simulink model "phasor08_ieee13_1_sm_master"  (Simulink 10.2)
settings: Solver=ode4  StartTime=0.0  StopTime=inf  FixedStep=0.01  RelTol=1e-3  EnableMultiTasking=on
PreLoadFcn:
  | Ts=0.01;
PostLoadFcn:
  | Ts=0.01;
InitFcn:
  | Ts=0.01;
StartFcn:
  | Ts=0.01;
libraries: opal_lib x5, eph_overcurrent x1, rtlab_phasor x1
settings Model: Creator=ZhiqiZhao  LastModifiedBy=xjk374
settings DataIOCC: LimitDataPoints=on
settings OptimizationCC: ExpressionDepthLimit=2147483647  LocalBlockOutputs=off
settings DebuggingCC: SolverPrmCheckMsg=warning  AllowSymbolicDim=off  StateNameClashWarn=warning
settings RTWCC: GenCodeOnly=on

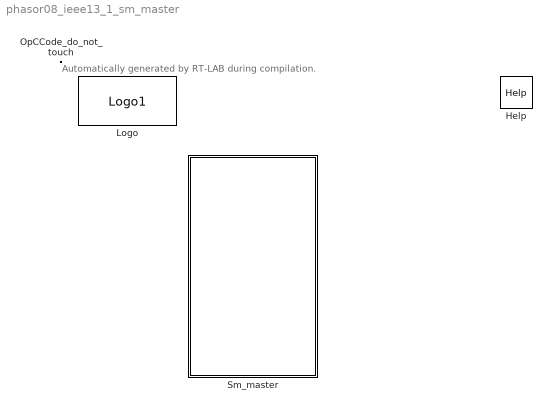
== system phasor08_ieee13_1_sm_master ==
  note: Automatically generated by RT-LAB during compilation.
  Help : opal_lib/Help  docfile=../help/ePH_IEEE13.html
  Logo : opal_lib/Logo1  vide=[]
  OpCCode_do_not_touch : opal_lib/Communication/OpCCode  SystemSampleTime=-1  VariantActivationTime=update diagram  Latency=0  AutoFrameSizeCalculation=off
  Sm_master : Subsystem

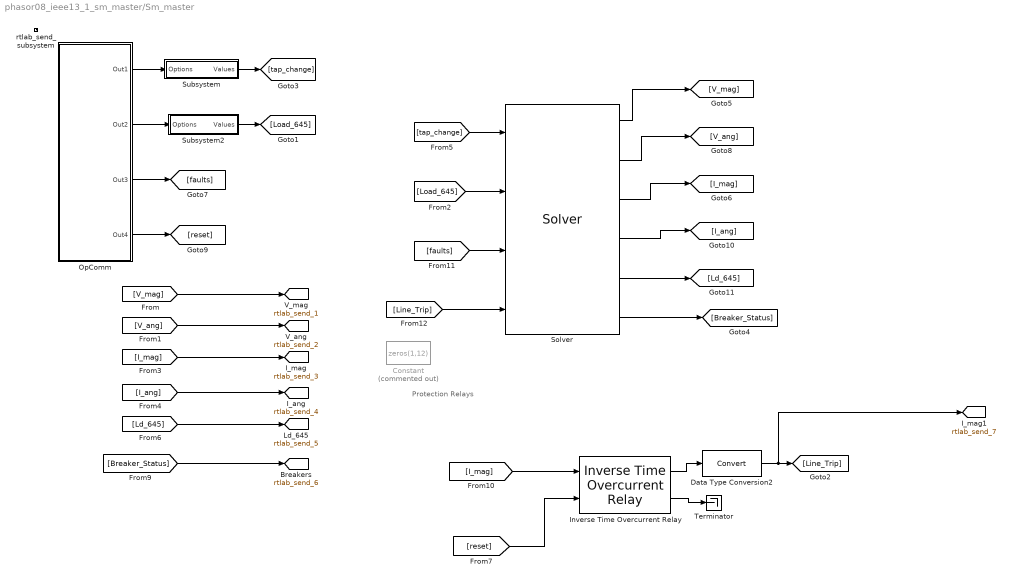
== system phasor08_ieee13_1_sm_master/Sm_master ==
  note: Protection
      | Relays
  Constant : Constant  Commented=on  Value=zeros(1,12)
  Data Type Conversion2 : DataTypeConversion
  Inverse Time Overcurrent Relay : eph_overcurrent/Inverse Time Overcurrent Relay  Ts=Ts  N=12  characteristic=6: I.E.C Class A - Standard inverse (0, 0.14, 0.02)  Ipck_51P=1000*ones(1,12)  TD51P=0.05*ones(1,12)
  OpComm : Subsystem
      mask init:
      | opmaskdisplay('maskdisplay_block',gcb,'disp(''OpComm'')');
      mask Display:
      | patch([0 0.5 0.7 0],[1 1 0 0],[0.7 0.75 0.9]);
      | patch([1 0.53 0.73 1],[1 1 0 0],[1 0.8 0.7]);
      | plot([0 0 1 1 0],[0 1 1 0 0]);
      | disp('OpComm')
  Solver : rtlab_phasor/Solver  epname=System  extension=Excel  use_udb=off  xls='phasor08_IEEE13.xls'  raw='4992b.raw'  dyr='4992b.dyr'  fmu2builtin=off  cyme='ieee13.sxst'  cyme_pf=''  cyme_unbalanced=on  powerfactory='network.xml'  builtin=on  lazy_netlist=on  capidir='CAPI'  fmudir=''  capiprefix=capicomp_  fmuprefix=fmucomp_  logging=off  sim_mode=Dynamic simulation only (without power-flow)  dt=Ts  pf_init_method=From input data  pf_tol_v=0.000001  pf_max_it=100  pf_smart_start=off  pf_flat_start=off  pf_export=off  pfrequest=off  pf_then_dyn=off  np=1  exporty=off  optim_threads=off  perflog_on=off  script_activate_postinit=off  script_postinit_name=''
  Subsystem : Subsystem
  Subsystem2 : Subsystem
  Terminator : Terminator
  rtlab_send_subsystem : Subsystem  Priority=-100
      mask Display: text(0,0,'');
  tag scope: rtlab_send_1=global, rtlab_send_2=global, rtlab_send_3=global, rtlab_send_4=global, rtlab_send_5=global, rtlab_send_6=global, rtlab_send_7=global
  wires:
  [tap_change] -> Solver/1
  Solver/1 -> [V_mag]
  Solver/2 -> [V_ang]
  Solver/3 -> [I_mag]
  Solver/4 -> [I_ang]
  Solver/5 -> [Ld_645]
  [Load_645] -> Solver/2
  [V_mag] -> [rtlab_send_1]
  [V_ang] -> [rtlab_send_2]
  [I_ang] -> [rtlab_send_4]
  [I_mag] -> [rtlab_send_3]
  [Ld_645] -> [rtlab_send_5]
  OpComm/1(Out1) -> Subsystem/1(Options)
  OpComm/2(Out2) -> Subsystem2/1(Options)
  Subsystem/1(Values) -> [tap_change]
  Subsystem2/1(Values) -> [Load_645]
  Inverse Time Overcurrent Relay/2 -> Terminator/1
  [reset] -> Inverse Time Overcurrent Relay/2
  Data Type Conversion2/1 -> [rtlab_send_7], [Line_Trip]
  Solver/6 -> [Breaker_Status]
  [Breaker_Status] -> [rtlab_send_6]
  Inverse Time Overcurrent Relay/1 -> Data Type Conversion2/1
  [I_mag] -> Inverse Time Overcurrent Relay/1
  OpComm/3(Out3) -> [faults]
  [faults] -> Solver/3
  [Line_Trip] -> Solver/4
  OpComm/4(Out4) -> [reset]

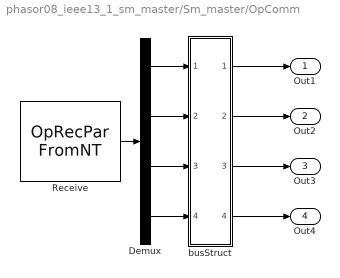
== system phasor08_ieee13_1_sm_master/Sm_master/OpComm ==
  Demux : Demux  Outputs="[7  5  4  1]"
  Receive : opal_lib/Communication/OpRecPar FromNT  Data_width=17  InitialConditions=[8;8;8;1;0;0;0;340;250;5;170;125;0;0;0;0;0]
  busStruct : Subsystem
  Out1 : Outport
  Out2 : Outport  Port=2
  Out3 : Outport  Port=3
  Out4 : Outport  Port=4
  wires:
  Demux/4 -> busStruct/4(In4)
  Demux/3 -> busStruct/3(In3)
  Demux/2 -> busStruct/2(In2)
  Demux/1 -> busStruct/1(In1)
  busStruct/4(Out4) -> Out4/1
  busStruct/3(Out3) -> Out3/1
  busStruct/2(Out2) -> Out2/1
  busStruct/1(Out1) -> Out1/1
  Receive/1 -> Demux/1

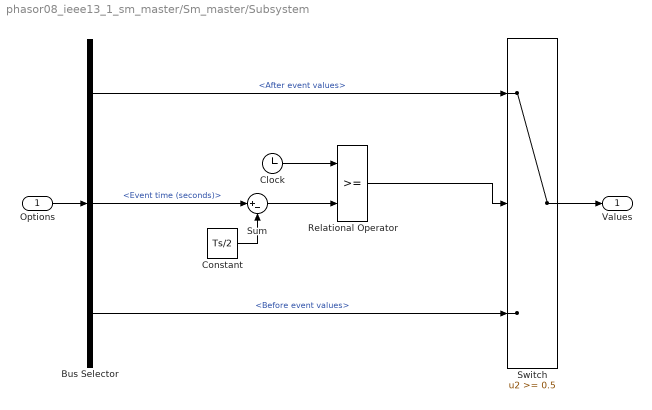
== system phasor08_ieee13_1_sm_master/Sm_master/Subsystem ==
  Options : Inport
  Bus Selector : BusSelector  OutputSignals=After event values,Event time (seconds),Before event values
  Clock : Clock
  Constant : Constant  Value=Ts/2
  Relational Operator : RelationalOperator  OutDataTypeStr=boolean  RndMeth=Nearest
  Sum : Sum  Inputs=|+-
  Switch : Switch  Threshold=0.5
  Values : Outport
  wires:
  Clock/1 -> Relational Operator/1
  Constant/1 -> Sum/2
  Sum/1 -> Relational Operator/2
  Bus Selector/2 -> Sum/1  "<Event time (seconds)>"
  Relational Operator/1 -> Switch/2
  Bus Selector/3 -> Switch/3  "<Before event values>"
  Bus Selector/1 -> Switch/1  "<After event values>"
  Switch/1 -> Values/1
  Options/1 -> Bus Selector/1

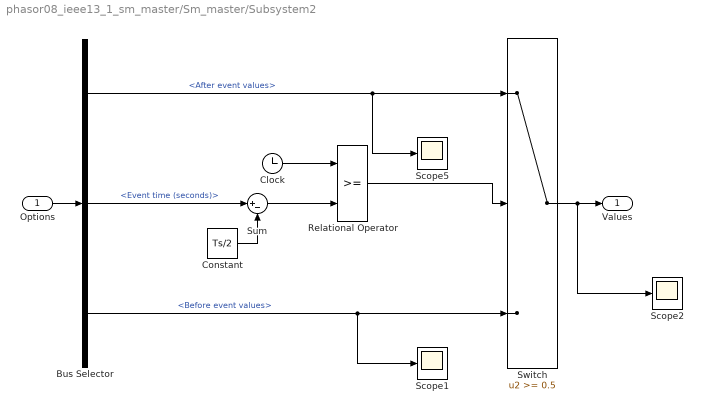
== system phasor08_ieee13_1_sm_master/Sm_master/Subsystem2 ==
  Options : Inport
  Bus Selector : BusSelector  OutputSignals=After event values,Event time (seconds),Before event values
  Clock : Clock
  Constant : Constant  Value=Ts/2
  Relational Operator : RelationalOperator  OutDataTypeStr=boolean  RndMeth=Nearest
  Scope1 : Scope
  Scope2 : Scope
  Scope5 : Scope
  Sum : Sum  Inputs=|+-
  Switch : Switch  Threshold=0.5
  Values : Outport
  wires:
  Clock/1 -> Relational Operator/1
  Constant/1 -> Sum/2
  Sum/1 -> Relational Operator/2
  Bus Selector/2 -> Sum/1  "<Event time (seconds)>"
  Relational Operator/1 -> Switch/2
  Bus Selector/3 -> Switch/3, Scope1/1  "<Before event values>"
  Bus Selector/1 -> Switch/1, Scope5/1  "<After event values>"
  Switch/1 -> Values/1, Scope2/1
  Options/1 -> Bus Selector/1

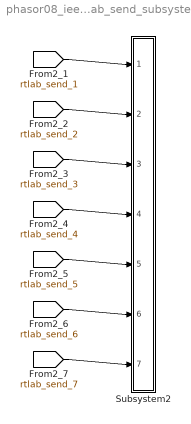
== system phasor08_ieee13_1_sm_master/Sm_master/rtlab_send_subsystem ==
  Subsystem2 : Subsystem
  wires:
  [rtlab_send_1] -> Subsystem2/1(In1)
  [rtlab_send_2] -> Subsystem2/2(In2)
  [rtlab_send_3] -> Subsystem2/3(In3)
  [rtlab_send_4] -> Subsystem2/4(In4)
  [rtlab_send_5] -> Subsystem2/5(In5)
  [rtlab_send_6] -> Subsystem2/6(In6)
  [rtlab_send_7] -> Subsystem2/7(In7)

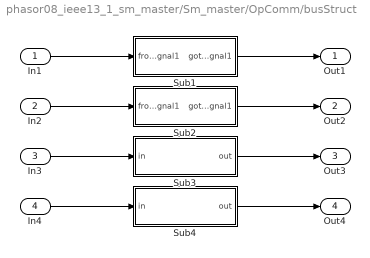
== system phasor08_ieee13_1_sm_master/Sm_master/OpComm/busStruct ==
  In1 : Inport
  In2 : Inport  Port=2
  In3 : Inport  Port=3
  In4 : Inport  Port=4
  Sub1 : Subsystem
  Sub2 : Subsystem
  Sub3 : Subsystem
  Sub4 : Subsystem
  Out1 : Outport
  Out2 : Outport  Port=2
  Out3 : Outport  Port=3
  Out4 : Outport  Port=4
  wires:
  Sub4/1(out) -> Out4/1
  In4/1 -> Sub4/1(in)
  Sub3/1(out) -> Out3/1
  In3/1 -> Sub3/1(in)
  Sub2/1(goto_signal1) -> Out2/1
  In2/1 -> Sub2/1(from_signal1)
  Sub1/1(goto_signal1) -> Out1/1
  In1/1 -> Sub1/1(from_signal1)

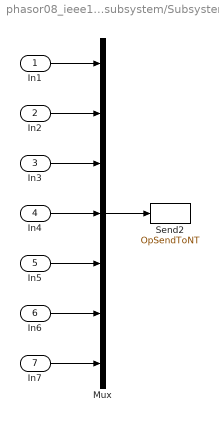
== system phasor08_ieee13_1_sm_master/Sm_master/rtlab_send_subsystem/Subsystem2 ==
  In1 : Inport
  In2 : Inport  Port=2
  In3 : Inport  Port=3
  In4 : Inport  Port=4
  In5 : Inport  Port=5
  In6 : Inport  Port=6
  In7 : Inport  Port=7
  Mux : Mux  Inputs=7
  Send2 : opal_lib/Communication/OpSendToNT  Acqu_group=1
  wires:
  Mux/1 -> Send2/1
  In1/1 -> Mux/1
  In2/1 -> Mux/2
  In3/1 -> Mux/3
  In4/1 -> Mux/4
  In5/1 -> Mux/5
  In6/1 -> Mux/6
  In7/1 -> Mux/7

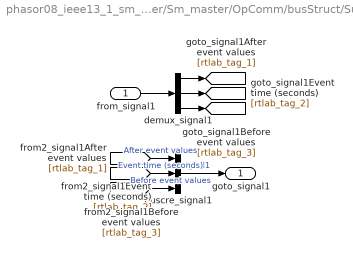
== system phasor08_ieee13_1_sm_master/Sm_master/OpComm/busStruct/Sub1 ==
  from_signal1 : Inport
  buscre_signal1 : BusCreator  Inputs=3
  demux_signal1 : Demux  Outputs="[3  1  3]"
  goto_signal1 : Outport
  wires:
  buscre_signal1/1 -> goto_signal1/1  "signal1"
  [rtlab_tag_3] -> buscre_signal1/3  "Before event values"
  [rtlab_tag_2] -> buscre_signal1/2  "Event time (seconds)"
  [rtlab_tag_1] -> buscre_signal1/1  "After event values"
  demux_signal1/3 -> [rtlab_tag_3]
  demux_signal1/2 -> [rtlab_tag_2]
  demux_signal1/1 -> [rtlab_tag_1]
  from_signal1/1 -> demux_signal1/1

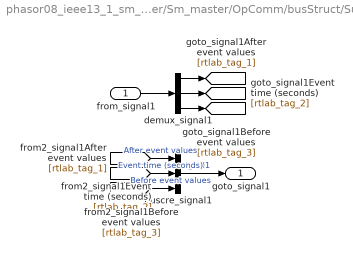
== system phasor08_ieee13_1_sm_master/Sm_master/OpComm/busStruct/Sub2 ==
  from_signal1 : Inport
  buscre_signal1 : BusCreator  Inputs=3
  demux_signal1 : Demux  Outputs="[2  1  2]"
  goto_signal1 : Outport
  wires:
  buscre_signal1/1 -> goto_signal1/1  "signal1"
  [rtlab_tag_3] -> buscre_signal1/3  "Before event values"
  [rtlab_tag_2] -> buscre_signal1/2  "Event time (seconds)"
  [rtlab_tag_1] -> buscre_signal1/1  "After event values"
  demux_signal1/3 -> [rtlab_tag_3]
  demux_signal1/2 -> [rtlab_tag_2]
  demux_signal1/1 -> [rtlab_tag_1]
  from_signal1/1 -> demux_signal1/1

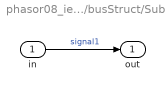
== system phasor08_ieee13_1_sm_master/Sm_master/OpComm/busStruct/Sub3 ==
  in : Inport
  out : Outport
  wires:
  in/1 -> out/1  "signal1"

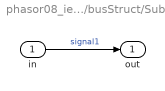
== system phasor08_ieee13_1_sm_master/Sm_master/OpComm/busStruct/Sub4 ==
  in : Inport
  out : Outport
  wires:
  in/1 -> out/1  "signal1"
